simulink model "nonlinear_closed_observer"  (R2024a)
settings: Solver=VariableStepAuto  StartTime=0.0  StopTime=15  MaxStep=1e-3  RelTol=1e-3
values from neighbouring files (symbols this model uses):
  A = [0, 1, 0, 0 ... (first row only)    [nonlinear_with_observer.m]    (also in nonlinear_with_reduced_observer.m; t_31.m; t_311.m; t_312.m)
  B = [0; J / ((M+m)*J - beta^2); 0; -beta / ((M+m)*J - beta^2)]    [nonlinear_with_observer.m]    (also in nonlinear_with_reduced_observer.m = [0; J/Delta0; 0; -beta/Delta0]; t_31.m = [0; J/Meff; 0; -beta/Meff]; t_311.m = [0; J/Meff; 0; -beta/Meff]; t_312.m = [0; J/Meff; 0; -beta/Meff])
  beta = m * lc    (= 40.0551)    [t_31.m]    (also in t_311.m; t_312.m; t_32.m; t_321.m)
  C = [1, 0, 0, 0 ... (first row only)    [nonlinear_with_observer.m]    (also in nonlinear_with_reduced_observer.m; t_31.m; t_311.m; t_312.m)
  f = 0    [nonlinear_model_closed.m]    (also in nonlinear_with_observer.m; nonlinear_with_reduced_observer.m; t_312.m; t_32.m)
  g = 9.81    [t_31.m]    (also in t_311.m; t_312.m; t_32.m; t_321.m)
  J = (1/3)*m1*l^2 + m2*l^2    (= 62.720658)    [t_31.m]    (also in t_311.m; t_312.m; t_32.m; t_321.m)
  K = [0 0 0 1] * inv(U) * D_A    [t_31.m]    (also in t_311.m = 1.0e+04*[-0.0046   -0.0233   -1.0984   -0.3688]; t_312.m = acker(A, B, lamJe); t_32.m = [-46.28, -233.21, -10984.45, -3688.10]; t_321.m = [-46.28, -233.21, -10984.45, -3688.10])
  L = place(A', C', lam_obs)'    [design_full_observer.m]    (also in t_32.m; t_321.m; t_33.m = [9.2705   -0.9852; t_331.m = place(A', C', L_spec)')
  M = 658.36    [t_31.m]    (also in t_311.m; t_312.m; t_32.m; t_321.m)
  m = m1 + m2    (= 30.46)    [t_31.m]    (also in t_311.m; t_312.m; t_32.m; t_321.m)
  x0 = x0_list{i}    [t_31.m]    (also in t_311.m; t_312.m = [0.1; 0.2; 0.03; 0.12]; t_32.m = [0.1; 0.2; 0.03; 0.12]; t_321.m = [0.1; 0.2; 0.03; 0.12])
settings Model: Creator=eva  LastModifiedBy=eva

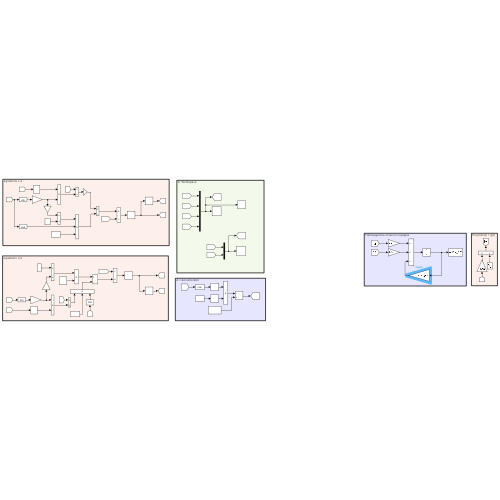
[thumbnail: Simulink's stored preview of the top-level diagram]
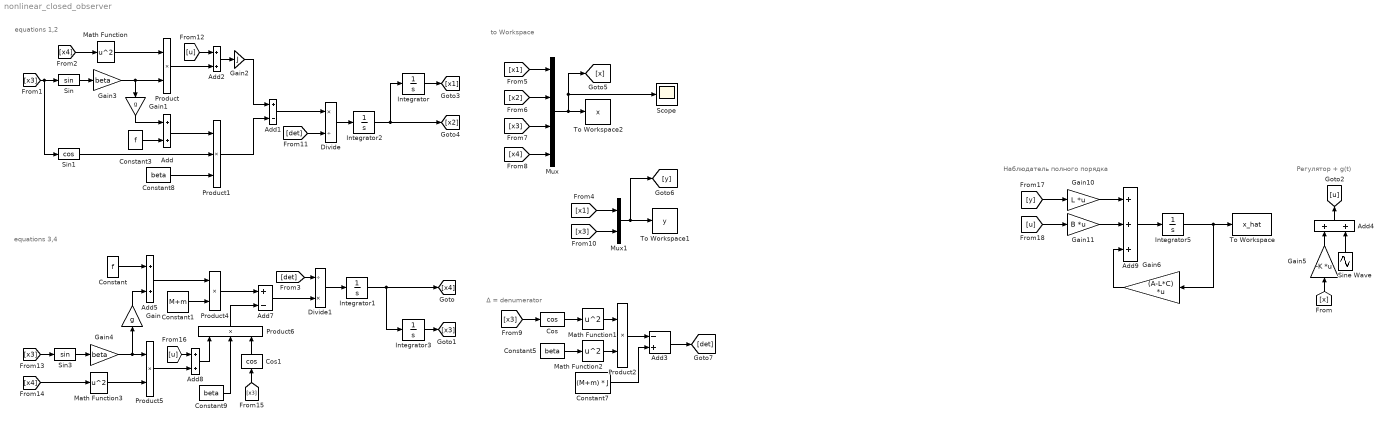
== system nonlinear_closed_observer ==
  note: Наблюдатель полного порядка
  note: equations 1,2
  note: Регулятор + g(t)
  note: equations 3,4
  note: to Workspace
  note: Δ = denumerator
  Add{,2,4..5,8} (5 alike) : Sum
  Add1 : Sum  Inputs=+-
  Add3 : Sum  Inputs=-+
  Add7 : Sum  Inputs=+-
  Add9 : Sum  Inputs=+++
  Constant : Constant  Value=f
  Constant1 : Constant  Value=M+m
  Constant3 : Constant  Value=f
  Constant5 : Constant  Value=beta
  Constant7 : Constant  Value=(M+m) * J
  Constant8 : Constant  Value=beta
  Constant9 : Constant  Value=beta
  Cos : Trigonometry  Operator=cos
  Cos1 : Trigonometry  Operator=cos
  Divide : Product  Inputs=*/
  Divide1 : Product  Inputs=/*
  Gain : Gain  Gain=g
  Gain1 : Gain  Gain=g
  Gain10 : Gain  Gain=L  Multiplication=Matrix(K*u)
  Gain11 : Gain  Gain=B  Multiplication=Matrix(K*u)
  Gain2 : Gain  Gain=J
  Gain3 : Gain  Gain=beta
  Gain4 : Gain  Gain=beta
  Gain5 : Gain  Gain=-K  Multiplication=Matrix(K*u)
  Gain6 : Gain  Gain=(A-L*C)  Multiplication=Matrix(K*u)
  Integrator : Integrator  InitialCondition=x0(1)
  Integrator1 : Integrator  InitialCondition=x0(4)
  Integrator2 : Integrator  InitialCondition=x0(2)
  Integrator3 : Integrator  InitialCondition=x0(3)
  Integrator5 : Integrator  InitialCondition=[0,0,0,0]
  Math Function{,1..3} (4 alike) : Math  Operator=square
  Mux : Mux
  Mux1 : Mux  Inputs=2
  Product{,2,4..5} (4 alike) : Product
  Product1 : Product  Inputs=3
  Product6 : Product  Inputs=3
  Scope : Scope
  Sin : Trigonometry
  Sin1 : Trigonometry  Operator=cos
  Sin3 : Trigonometry
  Sine Wave : Sin  Amplitude=2  Frequency=2  SampleTime=0
  To Workspace : ToWorkspace  VariableName=x_hat  SaveFormat=Structure With Time  SampleTime=-1
  To Workspace1 : ToWorkspace  VariableName=y  SaveFormat=Structure With Time  SampleTime=-1
  To Workspace2 : ToWorkspace  VariableName=x  SaveFormat=Structure With Time  SampleTime=-1
  wires:
  [x1] -> Mux/1
  [x3] -> Mux1/2
  Gain/1 -> Add5/2
  Constant/1 -> Add5/1
  [x3] -> Cos1/1
  Add5/1 -> Product4/1
  Mux/1 -> [x], Scope/1, To Workspace2/1
  Add/1 -> Product1/1
  Divide1/1 -> Integrator1/1
  Product/1 -> Add2/2
  Sin3/1 -> Gain4/1
  Add1/1 -> Divide/1
  Cos/1 -> Math Function1/1
  Integrator/1 -> [x1]
  Product2/1 -> Add3/1
  [u] -> Add2/1
  [x3] -> Sin/1, Sin1/1
  Product5/1 -> Add8/2
  Divide/1 -> Integrator2/1
  Gain3/1 -> Product/2, Gain1/1
  Constant5/1 -> Math Function2/1
  Add8/1 -> Product6/1
  Add3/1 -> [det]
  Product4/1 -> Add7/1
  Constant3/1 -> Add/2
  Constant1/1 -> Product4/2
  [x] -> Gain5/1
  [x3] -> Cos/1
  Math Function3/1 -> Product5/2
  Sin/1 -> Gain3/1
  Add2/1 -> Gain2/1
  Sin1/1 -> Product1/2
  Integrator1/1 -> [x4], Integrator3/1
  [det] -> Divide/2
  Product6/1 -> Add7/2
  [x3] -> Sin3/1
  [x1] -> Mux1/1
  Constant7/1 -> Add3/2
  Integrator3/1 -> [x3]
  [det] -> Divide1/1
  Math Function/1 -> Product/1
  Gain4/1 -> Product5/1, Gain/1
  Gain2/1 -> Add1/1
  Integrator2/1 -> [x2], Integrator/1
  Math Function2/1 -> Product2/2
  Gain1/1 -> Add/1
  Mux1/1 -> [y], To Workspace1/1
  [x3] -> Mux/3
  Cos1/1 -> Product6/3
  Add7/1 -> Divide1/2
  [x4] -> Mux/4
  [x4] -> Math Function3/1
  Math Function1/1 -> Product2/1
  Constant9/1 -> Product6/2
  Product1/1 -> Add1/2
  [x2] -> Mux/2
  Constant8/1 -> Product1/3
  [u] -> Add8/1
  [x4] -> Math Function/1
  [y] -> Gain10/1
  [u] -> Gain11/1
  Gain10/1 -> Add9/1
  Gain11/1 -> Add9/2
  Add9/1 -> Integrator5/1
  Gain6/1 -> Add9/3
  Integrator5/1 -> Gain6/1, To Workspace/1
  Add4/1 -> [u]
  Gain5/1 -> Add4/1
  Sine Wave/1 -> Add4/2
